simulink model "adaptivecontrol_via_backstepping"  (R2024b)
settings: Solver=FixedStepAuto  StartTime=0.0  StopTime=10  FixedStep=0.00001  RelTol=1e-3
values from neighbouring files (symbols this model uses):
  c = 1000    [script.m]
  k = 20000    [script.m]
  m = 300    [script.m]
settings Model: Creator=sueda  LastModifiedBy=sueda
settings DebuggingCC: UnderSpecifiedDimensionMsg=warning

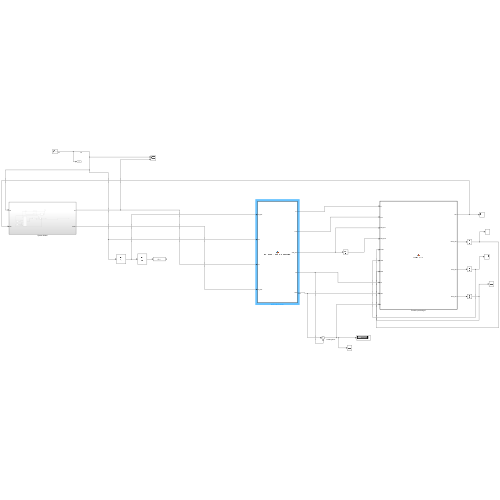
[thumbnail: Simulink's stored preview of the top-level diagram]
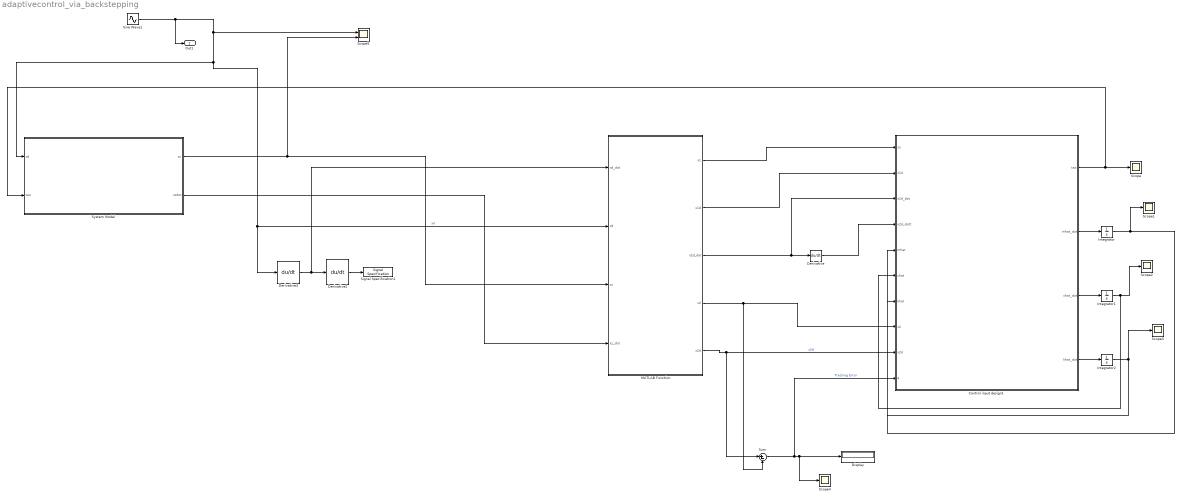
== system adaptivecontrol_via_backstepping ==
  Control input design1 : MATLAB Function  TreatAsAtomicUnit=on
  Derivative : Derivative
  Derivative2 : Derivative
  Derivative3 : Derivative
  Display : Display
  Integrator : Integrator
  Integrator1 : Integrator
  Integrator2 : Integrator
  MATLAB Function : MATLAB Function  TreatAsAtomicUnit=on
  Scope{,1..4} (5 alike) : Scope
  Scope5 : Scope  NumInputPorts=2
  Signal Specification1 : SignalSpecification  Dimensions=1
  Sine Wave1 : Sin  SampleTime=0
  Sum : Sum  Inputs=|+-
  System Model : Subsystem
  Out1 : Outport
  wires:
  Derivative3/1 -> MATLAB Function/1(xd_dot), Derivative2/1
  Derivative2/1 -> Signal Specification1/1
  Sine Wave1/1 -> Scope5/1, MATLAB Function/2(xd), Derivative3/1, System Model/1(xd), Out1/1  "xd"
  System Model/1(xz) -> Scope5/2, MATLAB Function/3(xz)
  System Model/2(xzdot) -> MATLAB Function/4(xz_dot)
  MATLAB Function/4(x2) -> Sum/2, Control input design1/8(x2)
  MATLAB Function/5(x2d) -> Sum/1, Control input design1/9(x2d)  "x2d"
  MATLAB Function/1(x1) -> Control input design1/1(x1)
  MATLAB Function/2(x1d) -> Control input design1/2(x1d)
  MATLAB Function/3(x2d_dot) -> Derivative/1, Control input design1/3(x2d_dot)
  Derivative/1 -> Control input design1/4(x2d_dott)
  Control input design1/2(mhat_dot) -> Integrator/1
  Control input design1/3(chat_dot) -> Integrator1/1
  Control input design1/4(khat_dot) -> Integrator2/1
  Integrator/1 -> Scope1/1, Control input design1/5(mhat)
  Integrator1/1 -> Scope2/1, Control input design1/6(chat)
  Integrator2/1 -> Scope3/1, Control input design1/7(khat)
  Control input design1/1(tao) -> System Model/2(tao), Scope/1
  Sum/1 -> Control input design1/10(e), Display/1, Scope4/1  "Tracking Error"

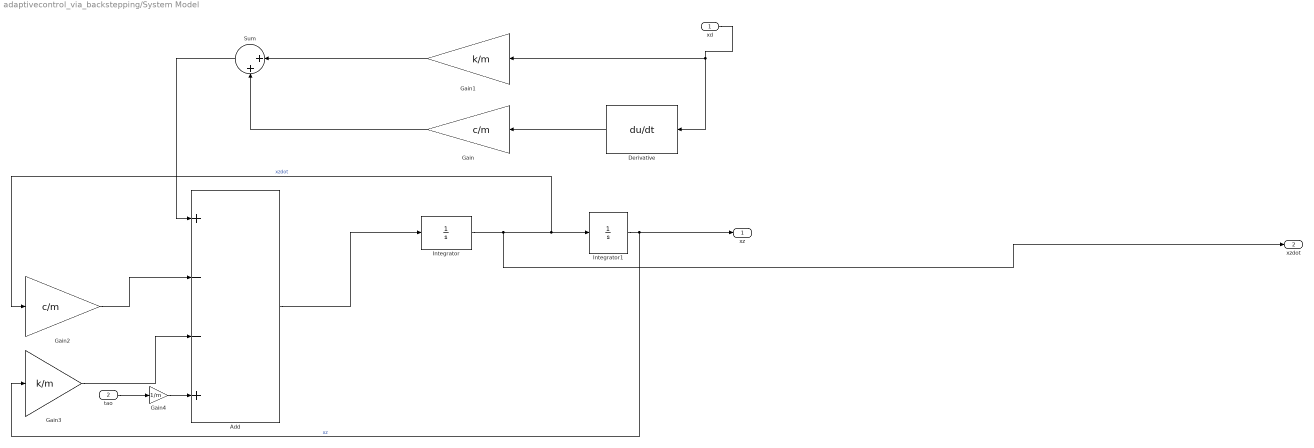
== system adaptivecontrol_via_backstepping/System Model ==
  xd : Inport
  tao : Inport  Port=2
  Add : Sum  Inputs=+--+
  Derivative : Derivative
  Gain : Gain  Gain=c/m
  Gain1 : Gain  Gain=k/m
  Gain2 : Gain  Gain=c/m
  Gain3 : Gain  Gain=k/m
  Gain4 : Gain  Gain=1/m
  Integrator : Integrator
  Integrator1 : Integrator
  Sum : Sum  Inputs=|++
  xz : Outport
  xzdot : Outport  Port=2
  wires:
  Integrator/1 -> xzdot/1, Integrator1/1, Gain2/1  "xzdot"
  xd/1 -> Derivative/1, Gain1/1
  Gain3/1 -> Add/3
  Integrator1/1 -> xz/1, Gain3/1  "xz"
  Gain2/1 -> Add/2
  Sum/1 -> Add/1
  Gain/1 -> Sum/2
  Gain1/1 -> Sum/1
  tao/1 -> Gain4/1
  Gain4/1 -> Add/4
  Add/1 -> Integrator/1
  Derivative/1 -> Gain/1

== matlab function adaptivecontrol_via_backstepping/MATLAB Function ==
  data: xd_dot input; x1 output; x1d output; x2d_dot output; x2 output; xd input; xz input; xz_dot input; x2d output
function [x1,x1d,x2d_dot,x2,x2d] = Backstepping_approach_parameters(xd_dot,xd,xz,xz_dot)

x1=xd_dot;
x2=xd;
x2_dot=x1;
x2d=xz;
x1d=xz_dot;
x2d_dot=x1d;

== matlab function adaptivecontrol_via_backstepping/Control input design1 ==
  data: x1 input; x1d input; x2d_dot input; x2d_dott input; mhat input; chat input; khat input; x2 input; x2d input; tao output; mhat_dot output; e input; chat_dot output; khat_dot output
function [tao,mhat_dot,chat_dot,khat_dot] = control_input(x1,x1d,x2d_dot,x2d_dott,mhat,chat,khat,x2,x2d,e)
    % Parameters
    m = 300;      % kg
    c = 1000;     % Ns/m
    k = 20000;    % N/m
    Kv= 9;
    Kg=10;
    
    %Error Definitions
    edot=-Kv*e;
    Uv=x2d_dot+Kv*e;
    ev=Uv-x1;
    %Lyapunov like stability analysis
    
    V1=1/2*e^2;
    V1_dot=-Kv*e^2;

    %Doing Stability Analysis i found mhat_dot,chat_dot and khat_dot
   
    mhat_dot=ev*(x2d_dott+Kv*edot);
    chat_dot=ev*(x1-x1d);
    khat_dot=ev*(x2-x2d);
    
    %Control Input tao Design
    tao=mhat*x2d_dott+mhat*Kv*edot+chat*(x1-x1d)+khat*(x2-x2d)+Kg*ev;
 
end
